simulink model "state_fb"  (Simulink 8.6)
settings: Solver=ode45  StartTime=0.0  StopTime=5  MaxStep=0.001  RelTol=1e-3
settings Model: Creator=Thomas Chmielewski  LastModifiedBy=DR_C
settings OptimizationCC: InitFltsAndDblsToZero=on
settings DebuggingCC: SaveWithParameterizedLinksMsg=none  SignalResolutionControl=TryResolveAllWithWarning  SolverPrmCheckMsg=none  MultiTaskDSMMsg=warning  MultiTaskCondExecSysMsg=none  FcnCallInpInsideContextMsg=UseLocalSettings
settings HardwareCC: TargetUnknown=on
settings GRTTargetCC: TargetFcnLib=ansi_tfl_tmw.mat  CompOptLevelCompliant=off

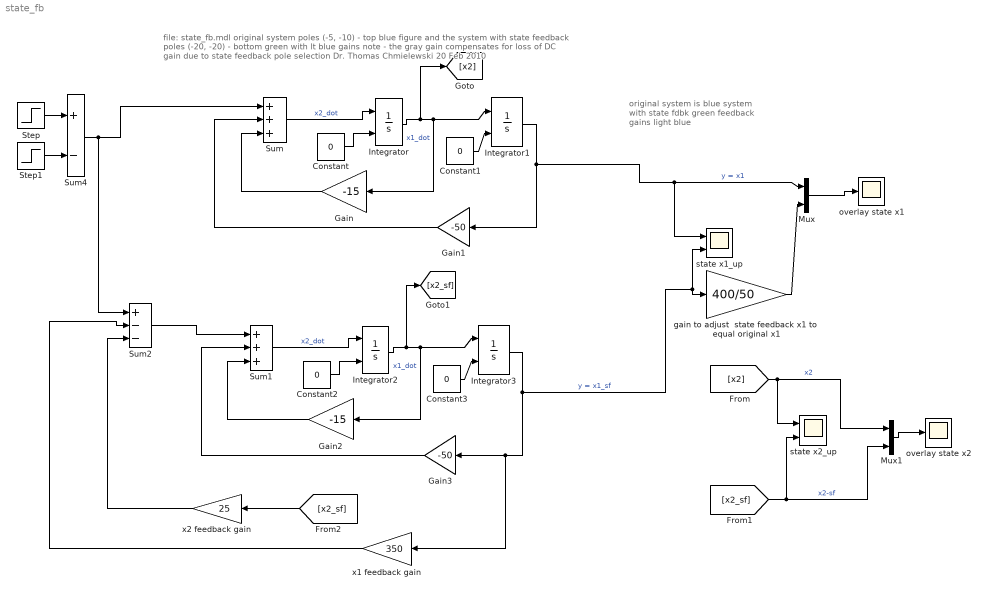
== system state_fb ==
  note: original system is blue
      | system with state fdbk green
      | feedback gains light blue
  note: file:  state_fb.mdl
      |  original system poles (-5, -10) - top blue figure
      | and the system with state feedback poles (-20, -20) - bottom green with lt blue gains
      | note - the gray gain compensates for loss of DC gain due to state feedback pole selection
      | Dr. Thomas Chmielewski 20 Feb 2010
  Constant{,1..3} (4 alike) : Constant  Value=0
  Gain : Gain  Gain=-15
  Gain1 : Gain  Gain=-50
  Gain2 : Gain  Gain=-15
  Gain3 : Gain  Gain=-50
  Integrator : Integrator  InitialConditionSource=external  InitialCondition=1
  Integrator1 : Integrator  InitialConditionSource=external  InitialCondition=10
  Integrator2 : Integrator  InitialConditionSource=external  InitialCondition=1
  Integrator3 : Integrator  InitialConditionSource=external  InitialCondition=10
  Mux : Mux  Inputs=2
  Mux1 : Mux  Inputs=2
  Step : Step  SampleTime=0
  Step1 : Step  Time=3  SampleTime=0
  Sum : Sum  Inputs=+++
  Sum1 : Sum  Inputs=+++
  Sum2 : Sum  Inputs=+--
  Sum4 : Sum  Inputs=+-
  gain to adjust  state feedback x1 to  equal original x1 : Gain  Gain=400/50
  overlay state x1 : Scope
  overlay state x2 : Scope
  state x1_up : Scope  NumInputPorts=2
  state x2_up : Scope  NumInputPorts=2
  x1 feedback gain : Gain  Gain=350
  x2 feedback gain : Gain  Gain=25
  wires:
  Integrator/1 -> Integrator1/1, Gain/1, [x2]  "x1_dot"
  Sum/1 -> Integrator/1  "x2_dot"
  Integrator1/1 -> Gain1/1, Mux/1, state x1_up/1  "y = x1"
  Gain/1 -> Sum/3
  Gain1/1 -> Sum/2
  Sum4/1 -> Sum2/1, Sum/1
  Step/1 -> Sum4/1
  Step1/1 -> Sum4/2
  Mux/1 -> overlay state x1/1
  Mux1/1 -> overlay state x2/1
  [x2] -> Mux1/1, state x2_up/1  "x2"
  [x2_sf] -> Mux1/2, state x2_up/2  "x2-sf"
  Constant/1 -> Integrator/2
  Constant1/1 -> Integrator1/2
  Integrator2/1 -> Integrator3/1, Gain2/1, [x2_sf]  "x1_dot"
  Sum1/1 -> Integrator2/1  "x2_dot"
  Integrator3/1 -> Gain3/1, x1 feedback gain/1, state x1_up/2, gain to adjust  state feedback x1 to  equal original x1/1  "y = x1_sf"
  Gain2/1 -> Sum1/3
  Gain3/1 -> Sum1/2
  Constant2/1 -> Integrator2/2
  Constant3/1 -> Integrator3/2
  Sum2/1 -> Sum1/1
  x2 feedback gain/1 -> Sum2/3
  x1 feedback gain/1 -> Sum2/2
  [x2_sf] -> x2 feedback gain/1
  gain to adjust  state feedback x1 to  equal original x1/1 -> Mux/2
